simulink library "CRYP_OLSERVO"  (Simulink 8.6)
settings: Solver=VariableStepAuto  StartTime=0.0  StopTime=10.0  RelTol=1e-3
libraries: cdsTP x48, cdsEpicsOut x48, cdsFiltCtrl x25, cdsEpicsStringIn x24, cdsRms x24, cdsFilt x24, cdsMuxMatrix x2, lockin x1
(part 1 of 4)
settings Model: Creator=controls  LastModifiedBy=controls

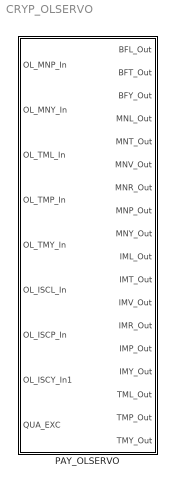
== system CRYP_OLSERVO ==
  PAY_OLSERVO : Subsystem

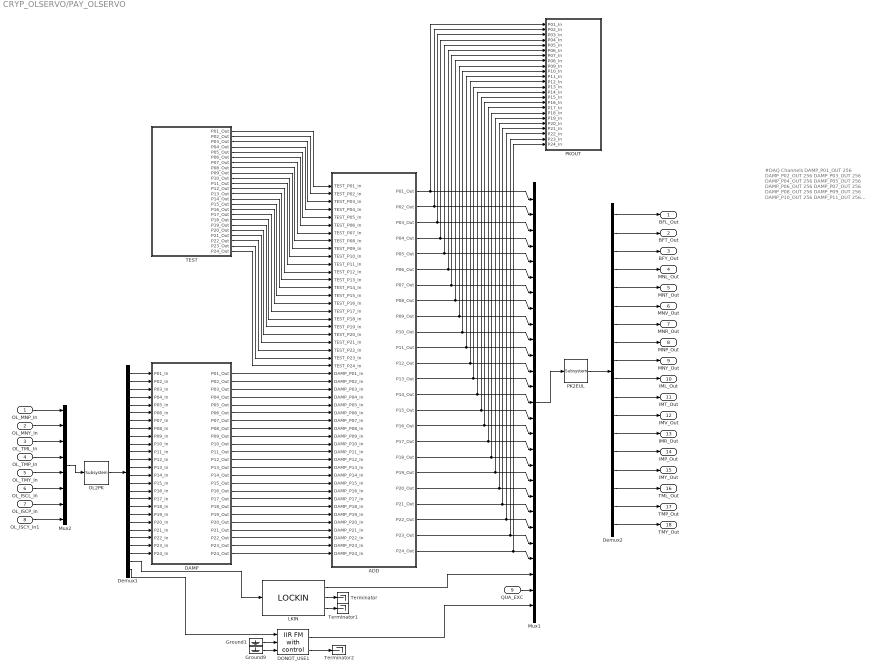
== system CRYP_OLSERVO/PAY_OLSERVO ==
  note: #DAQ Channels
      | DAMP_P01_OUT 256
      | DAMP_P02_OUT 256
      | DAMP_P03_OUT 256
      | DAMP_P04_OUT 256
      | DAMP_P05_OUT 256
      | DAMP_P06_OUT 256
      | DAMP_P07_OUT 256
      | DAMP_P08_OUT 256
      | DAMP_P09_OUT 256
      | DAMP_P10_OUT 256
      | DAMP_P11_OUT 256
      | DAMP_P12_OUT 256
      | DAMP_P13_OUT 256
      | DAMP_P14_OUT 256
      | DAMP_P15_OUT 256
      | DAMP_P16_OUT 256
      | DAMP_P17_OUT 256
      | DAMP_P18_OUT 256
      | DAMP_P19_OUT 256
      | DAMP_P20_OUT 256
      | DAMP_P21_OUT 256
      | DAMP_P22_OUT 256
      | DAMP_P23_OUT 256
      | DAMP_P24_OUT 256
      | LKIN_DEMOD_I_OUT 1024
      | LKIN_DEMOD_Q_OUT 1024
  OL_MNP_In : Inport
  OL_MNY_In : Inport  Port=2
  OL_TML_In : Inport  Port=3
  OL_TMP_In : Inport  Port=4
  OL_TMY_In : Inport  Port=5
  OL_ISCL_In : Inport  Port=6
  OL_ISCP_In : Inport  Port=7
  OL_ISCY_In1 : Inport  Port=8
  QUA_EXC : Inport  Port=9
  ADD : Subsystem
  DAMP : Subsystem
  DONOT_USE1 : cdsFiltCtrl/IIR FM with control  Tag=cdsFiltCtrl  Description=|
      | cdsFiltCntrl is the standard IIR filter module (exactly the same as cdsFilt) but with added control data output 'Ctrl'. Filter module digital signal output appears on the first output, which is called 'Val'. 'Ctrl' output has a bit pattern encoding the state of filter's on/off switches (FM1 through FM10). The bit values are:
      |                                                                                                                                                                                                                                                                                                                                       
      | module 	hex	dec                                                                                                                                                                                                                                                                                                                       
      | -----------------------                                                                                                                                                                                                                                                                                                               
      | FM1	0x20                    32                                                                                                                                                                                                                                                                                                        
      | FM2	0x80                     128                                                                                                                                                                                                                                                                                                      
      | FM3	0x200                   512                                                                                                                                                                                                                                                                                                       
      | FM4	0x800                   2048                                                                                                                                                                                                                                                                                                      
      | FM5	0x2000                 8192                                                                                                                                                                                                                                                                                                       
      | FM6	0x8000                 32768                                                                                                                                                                                                                                                                                                      
      | FM7	0x20000                131072                                                                                                                                                                                                                                                                                                     
      | FM8	0x80000                 524288                                                                                                                                                                                                                                                                                                    
      | FM9	0x200000               2097152                                                                                                                                                                                                                                                                                                    
      | FM10	0x800000               8388608                                                                                                                                                                                                                                                                                                   
      |                                                                                                                                                                                                                                                                                                                                       
      | This bit data can be used to drive some other switches or it can be output using a binary I/O module.
      settings: AttributesFormatString=%<Tag>
  Demux1 : Demux  Outputs=26
  Demux2 : Demux  Outputs=18
  Ground1 : Ground
  Ground9 : Ground
  LKIN : lockin/LOCKIN  Description=ADL=LOCKIN.adl
      settings: AttributesFormatString=%<Tag>
  Mux1 : Mux  Inputs=27
  Mux2 : Mux  Inputs=8
  OL2PK : cdsMuxMatrix/Subsystem  Tag=cdsMuxMatrix  Description=Any size matrix. Inputs and outputs must be connected using Mux and Demux parts.
      settings: AttributesFormatString=%<Tag>
  PK2EUL : cdsMuxMatrix/Subsystem  Tag=cdsMuxMatrix  Description=Any size matrix. Inputs and outputs must be connected using Mux and Demux parts.
      settings: AttributesFormatString=%<Tag>
  PKOUT : Subsystem
  TEST : Subsystem
  Terminator : Terminator
  Terminator1 : Terminator
  Terminator2 : Terminator
  BFL_Out : Outport
  BFT_Out : Outport  Port=2
  BFY_Out : Outport  Port=3
  MNL_Out : Outport  Port=4
  MNT_Out : Outport  Port=5
  MNV_Out : Outport  Port=6
  MNR_Out : Outport  Port=7
  MNP_Out : Outport  Port=8
  MNY_Out : Outport  Port=9
  IML_Out : Outport  Port=10
  IMT_Out : Outport  Port=11
  IMV_Out : Outport  Port=12
  IMR_Out : Outport  Port=13
  IMP_Out : Outport  Port=14
  IMY_Out : Outport  Port=15
  TML_Out : Outport  Port=16
  TMP_Out : Outport  Port=17
  TMY_Out : Outport  Port=18
  wires:
  DONOT_USE1/1 -> Mux1/27
  QUA_EXC/1 -> Mux1/26
  Demux1/26 -> DONOT_USE1/1
  Ground9/1 -> DONOT_USE1/3
  Ground1/1 -> DONOT_USE1/2
  DONOT_USE1/2 -> Terminator2/1
  LKIN/3 -> Terminator1/1
  LKIN/2 -> Terminator/1
  LKIN/1 -> Mux1/25
  Demux1/25 -> LKIN/1
  OL_ISCP_In/1 -> Mux2/7
  OL_ISCL_In/1 -> Mux2/6
  OL_TMP_In/1 -> Mux2/4
  OL_TMY_In/1 -> Mux2/5
  OL_MNP_In/1 -> Mux2/1
  OL_MNY_In/1 -> Mux2/2
  OL_TML_In/1 -> Mux2/3
  Mux2/1 -> OL2PK/1
  OL2PK/1 -> Demux1/1
  Demux1/3 -> DAMP/3(P03_In)
  Demux1/6 -> DAMP/6(P06_In)
  Demux1/4 -> DAMP/4(P04_In)
  Demux1/1 -> DAMP/1(P01_In)
  Demux1/2 -> DAMP/2(P02_In)
  Demux1/7 -> DAMP/7(P07_In)
  Demux1/8 -> DAMP/8(P08_In)
  Demux1/9 -> DAMP/9(P09_In)
  Demux1/10 -> DAMP/10(P10_In)
  Demux1/11 -> DAMP/11(P11_In)
  Demux1/12 -> DAMP/12(P12_In)
  Demux1/5 -> DAMP/5(P05_In)
  TEST/12(P12_Out) -> ADD/12(TEST_P12_In)
  TEST/6(P06_Out) -> ADD/6(TEST_P06_In)
  TEST/7(P07_Out) -> ADD/7(TEST_P07_In)
  TEST/8(P08_Out) -> ADD/8(TEST_P08_In)
  TEST/9(P09_Out) -> ADD/9(TEST_P09_In)
  TEST/10(P10_Out) -> ADD/10(TEST_P10_In)
  TEST/11(P11_Out) -> ADD/11(TEST_P11_In)
  TEST/1(P01_Out) -> ADD/1(TEST_P01_In)
  TEST/2(P02_Out) -> ADD/2(TEST_P02_In)
  TEST/3(P03_Out) -> ADD/3(TEST_P03_In)
  TEST/4(P04_Out) -> ADD/4(TEST_P04_In)
  TEST/5(P05_Out) -> ADD/5(TEST_P05_In)
  DAMP/11(P11_Out) -> ADD/35(DAMP_P11_In)
  DAMP/4(P04_Out) -> ADD/28(DAMP_P04_In)
  DAMP/5(P05_Out) -> ADD/29(DAMP_P05_In)
  DAMP/6(P06_Out) -> ADD/30(DAMP_P06_In)
  DAMP/12(P12_Out) -> ADD/36(DAMP_P12_In)
  DAMP/8(P08_Out) -> ADD/32(DAMP_P08_In)
  DAMP/10(P10_Out) -> ADD/34(DAMP_P10_In)
  DAMP/7(P07_Out) -> ADD/31(DAMP_P07_In)
  DAMP/9(P09_Out) -> ADD/33(DAMP_P09_In)
  DAMP/1(P01_Out) -> ADD/25(DAMP_P01_In)
  DAMP/2(P02_Out) -> ADD/26(DAMP_P02_In)
  DAMP/3(P03_Out) -> ADD/27(DAMP_P03_In)
  Mux1/1 -> PK2EUL/1
  PK2EUL/1 -> Demux2/1
  Demux1/13 -> DAMP/13(P13_In)
  Demux1/14 -> DAMP/14(P14_In)
  Demux1/15 -> DAMP/15(P15_In)
  Demux1/16 -> DAMP/16(P16_In)
  Demux1/17 -> DAMP/17(P17_In)
  Demux1/18 -> DAMP/18(P18_In)
  Demux1/19 -> DAMP/19(P19_In)
  Demux1/20 -> DAMP/20(P20_In)
  Demux1/21 -> DAMP/21(P21_In)
  Demux1/22 -> DAMP/22(P22_In)
  Demux1/23 -> DAMP/23(P23_In)
  Demux1/24 -> DAMP/24(P24_In)
  TEST/13(P13_Out) -> ADD/13(TEST_P13_In)
  TEST/14(P14_Out) -> ADD/14(TEST_P14_In)
  TEST/15(P15_Out) -> ADD/15(TEST_P15_In)
  TEST/16(P16_Out) -> ADD/16(TEST_P16_In)
  TEST/17(P17_Out) -> ADD/17(TEST_P17_In)
  TEST/18(P18_Out) -> ADD/18(TEST_P18_In)
  TEST/19(P19_Out) -> ADD/19(TEST_P19_In)
  TEST/20(P20_Out) -> ADD/20(TEST_P20_In)
  TEST/21(P21_Out) -> ADD/21(TEST_P21_In)
  TEST/22(P22_Out) -> ADD/22(TEST_P22_In)
  TEST/23(P23_Out) -> ADD/23(TEST_P23_In)
  TEST/24(P24_Out) -> ADD/24(TEST_P24_In)
  DAMP/13(P13_Out) -> ADD/37(DAMP_P13_In)
  DAMP/14(P14_Out) -> ADD/38(DAMP_P14_In)
  DAMP/15(P15_Out) -> ADD/39(DAMP_P15_In)
  DAMP/16(P16_Out) -> ADD/40(DAMP_P16_In)
  DAMP/17(P17_Out) -> ADD/41(DAMP_P17_In)
  DAMP/18(P18_Out) -> ADD/42(DAMP_P18_In)
  DAMP/19(P19_Out) -> ADD/43(DAMP_P19_In)
  DAMP/20(P20_Out) -> ADD/44(DAMP_P20_In)
  DAMP/21(P21_Out) -> ADD/45(DAMP_P21_In)
  DAMP/22(P22_Out) -> ADD/46(DAMP_P22_In)
  DAMP/23(P23_Out) -> ADD/47(DAMP_P23_In)
  DAMP/24(P24_Out) -> ADD/48(DAMP_P24_In)
  ADD/16(P16_Out) -> PKOUT/16(P16_In), Mux1/16
  ADD/14(P14_Out) -> PKOUT/14(P14_In), Mux1/14
  ADD/19(P19_Out) -> PKOUT/19(P19_In), Mux1/19
  ADD/20(P20_Out) -> PKOUT/20(P20_In), Mux1/20
  ADD/24(P24_Out) -> PKOUT/24(P24_In), Mux1/24
  ADD/22(P22_Out) -> PKOUT/22(P22_In), Mux1/22
  ADD/23(P23_Out) -> PKOUT/23(P23_In), Mux1/23
  ADD/13(P13_Out) -> PKOUT/13(P13_In), Mux1/13
  ADD/15(P15_Out) -> PKOUT/15(P15_In), Mux1/15
  ADD/2(P02_Out) -> PKOUT/2(P02_In), Mux1/2
  ADD/3(P03_Out) -> PKOUT/3(P03_In), Mux1/3
  ADD/4(P04_Out) -> PKOUT/4(P04_In), Mux1/4
  ADD/5(P05_Out) -> PKOUT/5(P05_In), Mux1/5
  ADD/6(P06_Out) -> PKOUT/6(P06_In), Mux1/6
  ADD/7(P07_Out) -> PKOUT/7(P07_In), Mux1/7
  ADD/8(P08_Out) -> PKOUT/8(P08_In), Mux1/8
  ADD/9(P09_Out) -> PKOUT/9(P09_In), Mux1/9
  ADD/10(P10_Out) -> PKOUT/10(P10_In), Mux1/10
  ADD/11(P11_Out) -> PKOUT/11(P11_In), Mux1/11
  ADD/12(P12_Out) -> PKOUT/12(P12_In), Mux1/12
  ADD/17(P17_Out) -> PKOUT/17(P17_In), Mux1/17
  ADD/18(P18_Out) -> PKOUT/18(P18_In), Mux1/18
  ADD/21(P21_Out) -> PKOUT/21(P21_In), Mux1/21
  ADD/1(P01_Out) -> PKOUT/1(P01_In), Mux1/1
  Demux2/1 -> BFL_Out/1
  Demux2/2 -> BFT_Out/1
  Demux2/3 -> BFY_Out/1
  Demux2/4 -> MNL_Out/1
  Demux2/5 -> MNT_Out/1
  Demux2/6 -> MNV_Out/1
  Demux2/7 -> MNR_Out/1
  Demux2/8 -> MNP_Out/1
  Demux2/9 -> MNY_Out/1
  Demux2/10 -> IML_Out/1
  Demux2/11 -> IMT_Out/1
  Demux2/12 -> IMV_Out/1
  Demux2/13 -> IMR_Out/1
  Demux2/14 -> IMP_Out/1
  Demux2/15 -> IMY_Out/1
  Demux2/16 -> TML_Out/1
  Demux2/18 -> TMY_Out/1
  Demux2/17 -> TMP_Out/1
  OL_ISCY_In1/1 -> Mux2/8

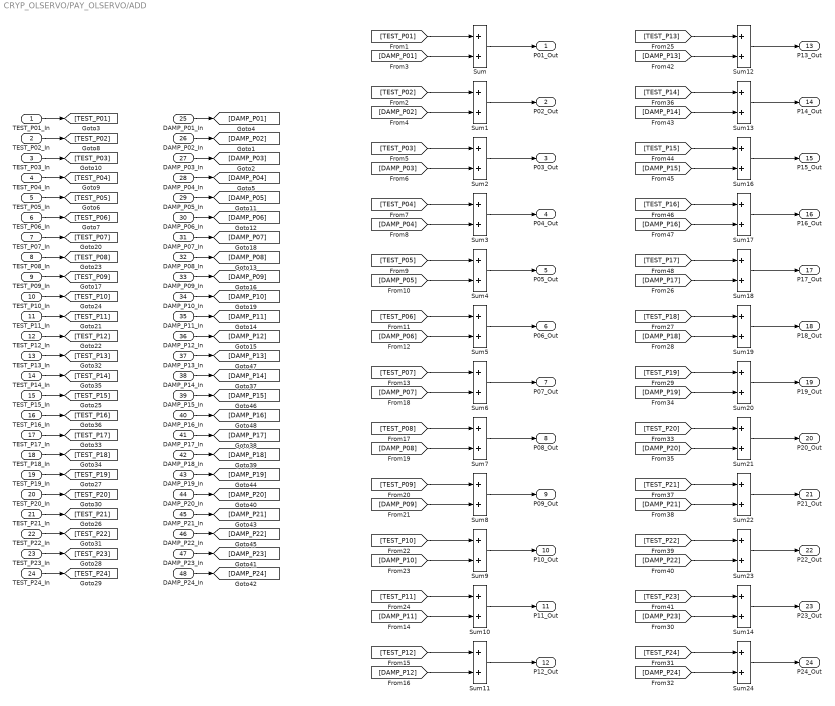
== system CRYP_OLSERVO/PAY_OLSERVO/ADD ==
  TEST_P01_In : Inport
  TEST_P02_In : Inport  Port=2
  TEST_P03_In : Inport  Port=3
  TEST_P04_In : Inport  Port=4
  TEST_P05_In : Inport  Port=5
  TEST_P06_In : Inport  Port=6
  TEST_P07_In : Inport  Port=7
  TEST_P08_In : Inport  Port=8
  TEST_P09_In : Inport  Port=9
  TEST_P10_In : Inport  Port=10
  TEST_P11_In : Inport  Port=11
  TEST_P12_In : Inport  Port=12
  TEST_P13_In : Inport  Port=13
  TEST_P14_In : Inport  Port=14
  TEST_P15_In : Inport  Port=15
  TEST_P16_In : Inport  Port=16
  TEST_P17_In : Inport  Port=17
  TEST_P18_In : Inport  Port=18
  TEST_P19_In : Inport  Port=19
  TEST_P20_In : Inport  Port=20
  TEST_P21_In : Inport  Port=21
  TEST_P22_In : Inport  Port=22
  TEST_P23_In : Inport  Port=23
  TEST_P24_In : Inport  Port=24
  DAMP_P01_In : Inport  Port=25
  DAMP_P02_In : Inport  Port=26
  DAMP_P03_In : Inport  Port=27
  DAMP_P04_In : Inport  Port=28
  DAMP_P05_In : Inport  Port=29
  DAMP_P06_In : Inport  Port=30
  DAMP_P07_In : Inport  Port=31
  DAMP_P08_In : Inport  Port=32
  DAMP_P09_In : Inport  Port=33
  DAMP_P10_In : Inport  Port=34
  DAMP_P11_In : Inport  Port=35
  DAMP_P12_In : Inport  Port=36
  DAMP_P13_In : Inport  Port=37
  DAMP_P14_In : Inport  Port=38
  DAMP_P15_In : Inport  Port=39
  DAMP_P16_In : Inport  Port=40
  DAMP_P17_In : Inport  Port=41
  DAMP_P18_In : Inport  Port=42
  DAMP_P19_In : Inport  Port=43
  DAMP_P20_In : Inport  Port=44
  DAMP_P21_In : Inport  Port=45
  DAMP_P22_In : Inport  Port=46
  DAMP_P23_In : Inport  Port=47
  DAMP_P24_In : Inport  Port=48
  Sum{,1..14,16..24} (24 alike) : Sum
  P01_Out : Outport
  P02_Out : Outport  Port=2
  P03_Out : Outport  Port=3
  P04_Out : Outport  Port=4
  P05_Out : Outport  Port=5
  P06_Out : Outport  Port=6
  P07_Out : Outport  Port=7
  P08_Out : Outport  Port=8
  P09_Out : Outport  Port=9
  P10_Out : Outport  Port=10
  P11_Out : Outport  Port=11
  P12_Out : Outport  Port=12
  P13_Out : Outport  Port=13
  P14_Out : Outport  Port=14
  P15_Out : Outport  Port=15
  P16_Out : Outport  Port=16
  P17_Out : Outport  Port=17
  P18_Out : Outport  Port=18
  P19_Out : Outport  Port=19
  P20_Out : Outport  Port=20
  P21_Out : Outport  Port=21
  P22_Out : Outport  Port=22
  P23_Out : Outport  Port=23
  P24_Out : Outport  Port=24
  wires:
  DAMP_P02_In/1 -> [DAMP_P02]
  DAMP_P01_In/1 -> [DAMP_P01]
  [DAMP_P01] -> Sum/2
  [TEST_P01] -> Sum/1
  Sum/1 -> P01_Out/1
  DAMP_P03_In/1 -> [DAMP_P03]
  TEST_P01_In/1 -> [TEST_P01]
  TEST_P02_In/1 -> [TEST_P02]
  TEST_P03_In/1 -> [TEST_P03]
  TEST_P04_In/1 -> [TEST_P04]
  TEST_P05_In/1 -> [TEST_P05]
  TEST_P06_In/1 -> [TEST_P06]
  DAMP_P05_In/1 -> [DAMP_P05]
  DAMP_P04_In/1 -> [DAMP_P04]
  DAMP_P06_In/1 -> [DAMP_P06]
  DAMP_P08_In/1 -> [DAMP_P08]
  DAMP_P07_In/1 -> [DAMP_P07]
  DAMP_P09_In/1 -> [DAMP_P09]
  DAMP_P11_In/1 -> [DAMP_P11]
  DAMP_P10_In/1 -> [DAMP_P10]
  DAMP_P12_In/1 -> [DAMP_P12]
  TEST_P07_In/1 -> [TEST_P07]
  TEST_P08_In/1 -> [TEST_P08]
  TEST_P09_In/1 -> [TEST_P09]
  TEST_P10_In/1 -> [TEST_P10]
  TEST_P11_In/1 -> [TEST_P11]
  TEST_P12_In/1 -> [TEST_P12]
  [DAMP_P02] -> Sum1/2
  [TEST_P02] -> Sum1/1
  Sum1/1 -> P02_Out/1
  [DAMP_P03] -> Sum2/2
  [TEST_P03] -> Sum2/1
  Sum2/1 -> P03_Out/1
  [DAMP_P04] -> Sum3/2
  [TEST_P04] -> Sum3/1
  Sum3/1 -> P04_Out/1
  [DAMP_P05] -> Sum4/2
  [TEST_P05] -> Sum4/1
  Sum4/1 -> P05_Out/1
  [DAMP_P06] -> Sum5/2
  [TEST_P06] -> Sum5/1
  Sum5/1 -> P06_Out/1
  [DAMP_P07] -> Sum6/2
  [TEST_P07] -> Sum6/1
  Sum6/1 -> P07_Out/1
  [DAMP_P08] -> Sum7/2
  [TEST_P08] -> Sum7/1
  Sum7/1 -> P08_Out/1
  [DAMP_P09] -> Sum8/2
  [TEST_P09] -> Sum8/1
  Sum8/1 -> P09_Out/1
  [DAMP_P10] -> Sum9/2
  [TEST_P10] -> Sum9/1
  Sum9/1 -> P10_Out/1
  [DAMP_P11] -> Sum10/2
  [TEST_P11] -> Sum10/1
  Sum10/1 -> P11_Out/1
  [DAMP_P12] -> Sum11/2
  [TEST_P12] -> Sum11/1
  Sum11/1 -> P12_Out/1
  TEST_P13_In/1 -> [TEST_P13]
  TEST_P14_In/1 -> [TEST_P14]
  TEST_P15_In/1 -> [TEST_P15]
  TEST_P16_In/1 -> [TEST_P16]
  TEST_P17_In/1 -> [TEST_P17]
  TEST_P18_In/1 -> [TEST_P18]
  TEST_P19_In/1 -> [TEST_P19]
  TEST_P20_In/1 -> [TEST_P20]
  TEST_P21_In/1 -> [TEST_P21]
  TEST_P22_In/1 -> [TEST_P22]
  TEST_P23_In/1 -> [TEST_P23]
  TEST_P24_In/1 -> [TEST_P24]
  DAMP_P14_In/1 -> [DAMP_P14]
  DAMP_P13_In/1 -> [DAMP_P13]
  DAMP_P15_In/1 -> [DAMP_P15]
  DAMP_P17_In/1 -> [DAMP_P17]
  DAMP_P16_In/1 -> [DAMP_P16]
  DAMP_P18_In/1 -> [DAMP_P18]
  DAMP_P20_In/1 -> [DAMP_P20]
  DAMP_P19_In/1 -> [DAMP_P19]
  DAMP_P21_In/1 -> [DAMP_P21]
  DAMP_P23_In/1 -> [DAMP_P23]
  DAMP_P22_In/1 -> [DAMP_P22]
  DAMP_P24_In/1 -> [DAMP_P24]
  [DAMP_P13] -> Sum12/2
  [TEST_P13] -> Sum12/1
  Sum12/1 -> P13_Out/1
  [DAMP_P14] -> Sum13/2
  [TEST_P14] -> Sum13/1
  Sum13/1 -> P14_Out/1
  [DAMP_P15] -> Sum16/2
  [TEST_P15] -> Sum16/1
  Sum16/1 -> P15_Out/1
  [DAMP_P16] -> Sum17/2
  [TEST_P16] -> Sum17/1
  Sum17/1 -> P16_Out/1
  [DAMP_P17] -> Sum18/2
  [TEST_P17] -> Sum18/1
  Sum18/1 -> P17_Out/1
  [DAMP_P18] -> Sum19/2
  [TEST_P18] -> Sum19/1
  Sum19/1 -> P18_Out/1
  [DAMP_P19] -> Sum20/2
  [TEST_P19] -> Sum20/1
  Sum20/1 -> P19_Out/1
  [DAMP_P20] -> Sum21/2
  [TEST_P20] -> Sum21/1
  Sum21/1 -> P20_Out/1
  [DAMP_P21] -> Sum22/2
  [TEST_P21] -> Sum22/1
  Sum22/1 -> P21_Out/1
  [DAMP_P22] -> Sum23/2
  [TEST_P22] -> Sum23/1
  Sum23/1 -> P22_Out/1
  [DAMP_P23] -> Sum14/2
  [TEST_P23] -> Sum14/1
  Sum14/1 -> P23_Out/1
  [DAMP_P24] -> Sum24/2
  [TEST_P24] -> Sum24/1
  Sum24/1 -> P24_Out/1
